simulink model "Quadruped_Plant"  (R2022b)
settings: Solver=VariableStepAuto  StartTime=0.0  StopTime=0.2  RelTol=1e-3
settings Model: Creator=papaveneti  LastModifiedBy=papaveneti

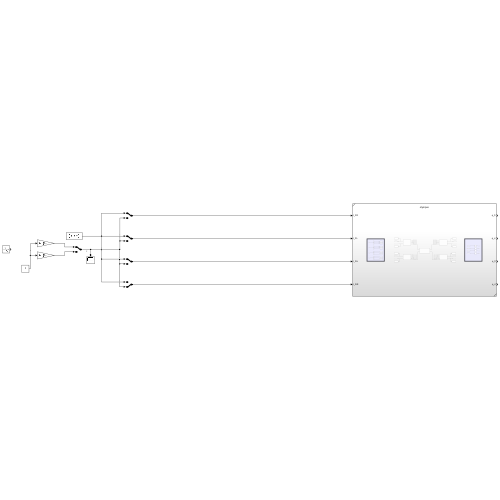
[thumbnail: Simulink's stored preview of the top-level diagram]
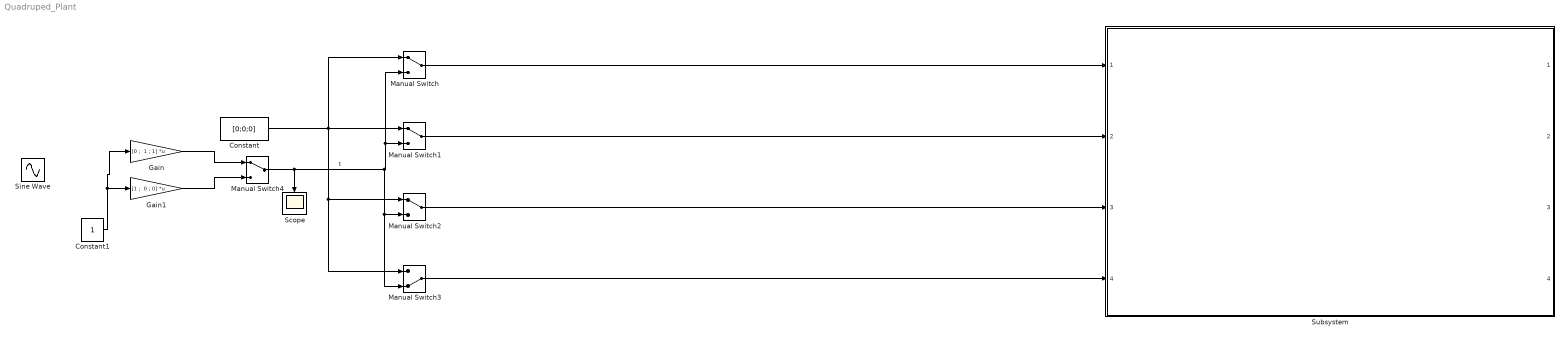
== system Quadruped_Plant ==
  Constant : Constant  Value=[0;0;0]
  Constant1 : Constant
  Gain : Gain  Gain="[0 ;  1 ; 1]"  Multiplication=Matrix(K*u)
  Gain1 : Gain  Gain="[1 ;  0 ; 0]"  Multiplication=Matrix(K*u)
  Manual Switch{,1..2,4} (4 alike) : ManualSwitch
  Manual Switch3 : ManualSwitch  CurrentSetting=0
  Scope : Scope
  Sine Wave : Sin  Amplitude=0.1  Frequency=2*pi/0.5  SampleTime=0
  Subsystem : Subsystem  ReferencedSubsystem=olympus
  wires:
  Manual Switch/1 -> Subsystem/1
  Manual Switch1/1 -> Subsystem/2
  Manual Switch2/1 -> Subsystem/3
  Manual Switch3/1 -> Subsystem/4
  Constant/1 -> Manual Switch/1, Manual Switch1/1, Manual Switch3/1, Manual Switch2/1
  Constant1/1 -> Gain/1, Gain1/1
  Manual Switch4/1 -> Scope/1, Manual Switch3/2, Manual Switch2/2, Manual Switch/2, Manual Switch1/2  "t"
  Gain/1 -> Manual Switch4/1
  Gain1/1 -> Manual Switch4/2
